simulink model "tmp"  (Simulink 7.4)
settings: Solver=ode45  StartTime=0  StopTime=1  FixedStep=ts  MaxStep=0.01  RelTol=1e-3
model workspace (MAT data in the model file):
  ts : num (value not decoded)
undefined symbols (not defined in the file): wing
libraries: simulink x2, cstblocks x1
settings Model: Creator=Rafal  ModifiedByFormat=Rafal  LastModifiedBy=Rafal  ModifiedComment=Rafal -- Sat Aug 10 21:22:15 2013 -- Version 1.359  ExtModeArmWhenConnect=off  BufferReuse=off
settings Model: ModifiedHistory=|
  | Rafal -- Sat Aug 10 21:22:15 2013 -- Version 1.359
  | 
  | 
  | Rafal -- Sat Aug 10 19:42:02 2013 -- Version 1.358
  | 
  | 
  | Rafal -- Sat Aug 10 19:16:36 2013 -- Version 1.357
  | 
  | 
  | Rafal -- Tue Jul 23 23:50:04 2013 -- Version 1.356
  | 
  | 
  | Rafal -- Sun Jul 21 15:07:54 2013 -- Version 1.355
  | 
  | 
  | Rafal -- Sun Jul 21 15:03:56 2013 -- Version 1.354
  | 
  | 
  | Rafal -- Sun Jul 21 14:29:27 2013 -- Version 1.353
  | 
  | 
  | Rafal -- Sun Jul 21 14:26:43 2013 -- Version 1.352
  | 
  | 
  | Rafal -- Sun Jul 21 14:20:01 2013 -- Version 1.351
  | 
  | 
  | Rafal -- Sun Jul 21 12:56:02 2013 -- Version 1.350
  | 
  | 
  | Rafal -- Sun Jul 21 12:54:49 2013 -- Version 1.349
  | 
  | 
  | Rafal -- Sun Jul 21 12:47:56 2013 -- Version 1.348
  | Regulator added
  | 
  | Rafal -- Tue Apr 23 17:26:44 2013 -- Version 1.347
  | 
  | 
  | Rafal -- Sat Feb 23 17:53:04 2013 -- Version 1.346
  | Turbulence applied directly to alpha calculation (not U0)
  | 
  | Rafal -- Sat Feb 23 17:44:49 2013 -- Version 1.345
  | Fix turbulence
  | 
  | Rafal -- Sat Feb 23 17:32:06 2013 -- Version 1.344
  | Turbulence. Only w is used (not w_dot)
  | 
  | Rafal -- Sat Feb 23 17:22:58 2013 -- Version 1.343
  | Turbulence added
  | 
  | Rafal -- Thu Feb 07 20:03:51 2013 -- Version 1.342
  | 
  | 
  | Rafal -- Thu Feb 07 20:02:41 2013 -- Version 1.341
  | 
  | 
  | Rafal -- Thu Feb 07 20:01:15 2013 -- Version 1.340
  | 
  | 
  | Rafal -- Thu Feb 07 19:10:07 2013 -- Version 1.339
  | Mask Wing subystem
  | 
  | Rafal -- Thu Feb 07 19:00:08 2013 -- Version 1.338
  | Wing subsystem moved to shared library
  | 
  | Rafal -- Thu Feb 07 18:59:31 2013 -- Version 1.337
  | Wing subsystem removed to shared library
  | 
  | Rafal -- Tue Feb 05 00:13:44 2013 -- Version 1.336
  | 
  | 
  | Rafal -- Tue Feb 05 00:12:22 2013 -- Version 1.335
  | 
  | 
  | Rafal -- Mon Feb 04 19:51:08 2013 -- Version 1.334
  | 
  | 
  | Rafal -- Mon Feb 04 19:14:36 2013 -- Version 1.333
  | 
  | 
  | Rafal -- Mon Feb 04 19:09:34 2013 -- Version 1.332
  | 
  | 
  | Rafal -- Mon Feb 04 19:01:45 2013 -- Version 1.331
  | 
  | 
  | Rafal -- Mon Feb 04 18:55:54 2013 -- Version 1.330
  | 
  | 
  | Rafal -- Mon Feb 04 18:24:17 2013 -- Version 1.329
  | 
  | 
  | Rafal -- Mon Feb 04 18:17:49 2013 -- Version 1.328
  | 
  | 
  | Rafal -- Mon Feb 04 02:04:22 2013 -- Version 1.327
  | 
  | 
  | Rafal -- Mon Feb 04 02:00:31 2013 -- Version 1.326
  | 
  | 
  | Rafal -- Mon Feb 04 01:01:05 2013 -- Version 1.325
  | 
  | 
  | Rafal -- Mon Feb 04 00:56:31 2013 -- Version 1.324
  | 
  | 
  | Rafal -- Mon Feb 04 00:48:55 2013 -- Version 1.323
  | SimRunner
  | 
  | Rafal -- Sun Feb 03 22:29:11 2013 -- Version 1.322
  | 
  | 
  | Rafal -- Sun Feb 03 22:11:10 2013 -- Version 1.321
  | 
  | 
  | Rafal -- Sun Feb 03 22:09:23 2013 -- Version 1.320
  | No initFcn
  | 
  | Rafal -- Fri Feb 01 00:20:34 2013 -- Version 1.319
  | 
  | 
  | Rafal -- Thu Jan 31 23:56:09 2013 -- Version 1.318
  | 
  | 
  | Rafal -- Thu Jan 31 23:45:26 2013 -- Version 1.317
  | 
  | 
  | Rafal -- Thu Jan 31 23:37:18 2013 -- Version 1.316
  | 
  | 
  | Rafal -- Thu Jan 31 23:32:50 2013 -- Version 1.315
  | 
  | 
  | Rafal -- Thu Jan 31 23:31:24 2013 -- Version 1.314
  | 
  | 
  | Rafal -- Sun Jan 20 23:13:45 2013 -- Version 1.313
  | Korzystamy z zewnetrznych parametrow bactParams, dumpBact
  | Dla danych z BACT wyniki pokrywaja sie idealnie z modelem analitycznym i modelem z Matlab files exchange
  | 
  | Rafal -- Sun Jan 20 20:08:58 2013 -- Version 1.312
  | 
  | 
  | Rafal -- Sun Jan 20 20:07:59 2013 -- Version 1.311
  | 
  | 
  | Rafal -- Sun Jan 20 20:04:53 2013 -- Version 1.310
  | 
  | 
  | Rafal -- Sun Jan 20 19:07:50 2013 -- Version 1.309
  | 
  | 
  | Rafal -- Sun Jan 20 18:53:01 2013 -- Version 1.308
  | 
  | 
  | Rafal -- Fri Jan 18 13:35:31 2013 -- Version 1.307
  | 
  | 
  | Rafal -- Thu Jan 17 00:20:40 2013 -- Version 1.306
  | 
  | 
  | Rafal -- Wed Jan 16 23:53:54 2013 -- Version 1.305
  | 
  | 
  | Rafal -- Wed Jan 16 23:42:52 2013 -- Version 1.304
  | Dodana konfiguracjaL CriticalSpeed do oszacowania predkosci krytycznej.
  | 
  | Rafal -- Wed Jan 16 19:50:35 2013 -- Version 1.303
  | Fix na linearyzacje.
  | Wczesniej Alpha_dot =  Alpha -> du/dt
  | Teraz:
  | Wywalony bloczek 'du/dt'.
  | Alpha_dot = Theta_dot - H_dot_dot/U0
  | Pochodna h_dot_dot wzieta bezposrednio z bloczku Wing Body
  | 
  | Rafal -- Wed Jan 16 15:02:06 2013 -- Version 1.302
  | 
  | 
  | Rafal -- Wed Jan 16 11:27:09 2013 -- Version 1.301
  | Turbulence addedd
settings DataIOCC: InitialState=simState  LimitDataPoints=off  SaveOutput=off  SignalLogging=off  SaveTime=off  SignalLoggingName=sigsOut
settings OptimizationCC: BlockReduction=off  InlineParams=on  OptimizeBlockIOStorage=off  BufferReuse=off  EnforceIntegerDowncast=off  ExpressionFolding=off  FoldNonRolledExpr=off  LocalBlockOutputs=off  InitFltsAndDblsToZero=on
settings DebuggingCC: AlgebraicLoopMsg=none  SaveWithParameterizedLinksMsg=none  SignalResolutionControl=TryResolveAllWithWarning  SolverPrmCheckMsg=none  MultiTaskDSMMsg=warning  MultiTaskCondExecSysMsg=none  UnconnectedInputMsg=none  UnconnectedOutputMsg=none  UnconnectedLineMsg=none  StrictBusMsg=None
settings HardwareCC: TargetUnknown=on
settings RTWCC: SystemTargetFile=xpctarget.tlc  TemplateMakefile=xpc_default_tmf  ProcessScript=xpctarget_make_rtw_hook  IncludeERTFirstTime=on
settings TargetCC: TargetFcnLib=ansi_tfl_tmw.mat  TargetFunctionLibrary=ANSI_C  IsPILTarget=off  CompOptLevelCompliant=off  MatFileLogging=on  EnableShiftOperators=on  PortableWordSizes=off
settings CustomProperty: DataType=string  Value=Real-Time
settings SimscapeCC: SelectedTab=SimMechanics

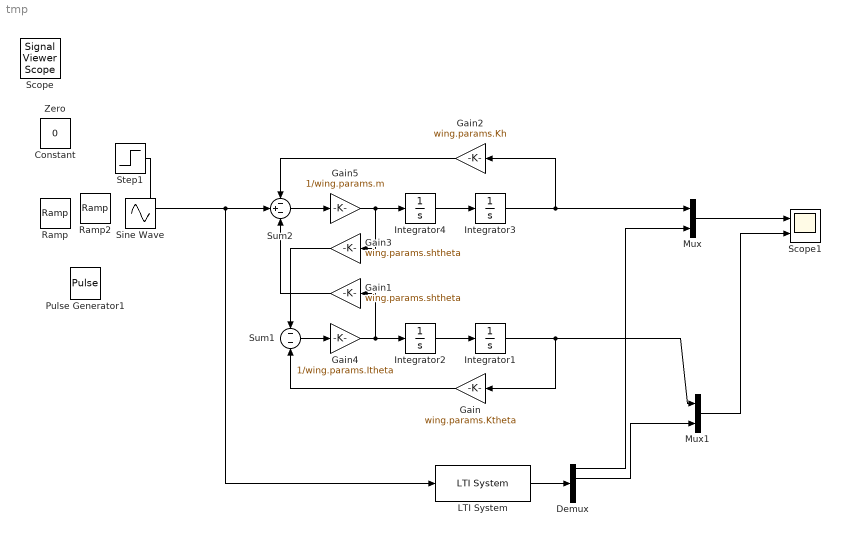
== system tmp ==
  Demux : Demux
  Gain : Gain  Gain=wing.params.Ktheta  ParameterDataType=fixdt(1, 16)  ParameterScaling=2^0  OutDataType=fixdt(1, 16)  OutScaling=2^0
  Gain1 : Gain  Gain=wing.params.shtheta  ParameterDataType=fixdt(1, 16)  ParameterScaling=2^0  OutDataType=fixdt(1, 16)  OutScaling=2^0
  Gain2 : Gain  Gain=wing.params.Kh  ParameterDataType=fixdt(1, 16)  ParameterScaling=2^0  OutDataType=fixdt(1, 16)  OutScaling=2^0
  Gain3 : Gain  Gain=wing.params.shtheta  ParameterDataType=fixdt(1, 16)  ParameterScaling=2^0  OutDataType=fixdt(1, 16)  OutScaling=2^0
  Gain4 : Gain  Gain=1/wing.params.Itheta  ParameterDataType=fixdt(1, 16)  ParameterScaling=2^0  OutDataType=fixdt(1, 16)  OutScaling=2^0
  Gain5 : Gain  Gain=1/wing.params.m  ParameterDataType=fixdt(1, 16)  ParameterScaling=2^0  OutDataType=fixdt(1, 16)  OutScaling=2^0
  Integrator{1..4} (4 alike) : Integrator
  LTI System : cstblocks/LTI System  SystemSampleTime=-1  sys=sys  IC=[]
  Mux : Mux  Inputs=2
  Mux1 : Mux  Inputs=2
  Pulse Generator1 : DiscretePulseGenerator  PulseType=Time based  Amplitude=1  Period=1  PulseWidth=5  PhaseDelay=0  SampleTime=1
  Ramp2 : simulink/Sources/Ramp  SystemSampleTime=-1  slope=1  start=0  X0=0
  Scope1 : Scope  NumInputPorts=2
      settings: YMin=-5~-5  YMax=5~5
  Step1 : Step  Time=0  SampleTime=0
  Sum1 : Sum  Inputs=-|-  OutDataType=fixdt(1, 16)  OutScaling=2^0
  Sum2 : Sum  Inputs=-+-  OutDataType=fixdt(1, 16)  OutScaling=2^0
  Constant : Constant  IOType=siggen  Value=-1  OutDataType=sfix(16)  OutScaling=2^0
  Ramp : simulink/Sources/Ramp  IOType=siggen  SystemSampleTime=-1  slope=1  start=0  X0=0
  Scope : SignalViewerScope  IOType=viewer  ZoomMode=xonly  LegendLocations="674.3333      275.3333            95            41"  RefreshTime=0.035000
      settings: ShowLegends=on  YMin=-0.0018  YMax=0.0002
  Sine Wave : Sin  IOType=siggen  Amplitude=10  Bias=0  Frequency=5  Phase=pi/2  Samples=10  SampleTime=0  Offset=0
  Zero : Constant  IOType=siggen  Value=0  OutDataType=sfix(16)  OutScaling=2^0
  wires:
  Integrator2/1 -> Integrator1/1
  Integrator1/1 -> Gain/1, Mux1/1
  Integrator4/1 -> Integrator3/1
  Integrator3/1 -> Gain2/1, Mux/1
  Gain2/1 -> Sum2/1
  Gain/1 -> Sum1/2
  Step1/1 -> Sum2/2, LTI System/1
  Sum1/1 -> Gain4/1
  Gain4/1 -> Integrator2/1, Gain1/1
  Sum2/1 -> Gain5/1
  Gain5/1 -> Integrator4/1, Gain3/1
  Gain3/1 -> Sum1/1
  Mux/1 -> Scope1/1
  LTI System/1 -> Demux/1
  Demux/1 -> Mux/2
  Mux1/1 -> Scope1/2
  Demux/2 -> Mux1/2
  Gain1/1 -> Sum2/3
